simulink model "moon_riders"  (R2023a)
settings: Solver=FixedStepDiscrete  StartTime=0.0  StopTime=10.0  FixedStep=0.1  RelTol=1e-3
settings Model: Creator=Roger  LastModifiedBy=Roger
settings OptimizationCC: DefaultParameterBehavior=Inlined  EnhancedBackFolding=on  PassReuseOutputArgsAs=Individual arguments  ZeroExternalMemoryAtStartup=off  ZeroInternalMemoryAtStartup=off  OptimizeBlockOrder=speed  DifferentSizesBufferReuse=on  OptimizationCustomize=off  EfficientTunableParamExpr=on
settings DebuggingCC: ParameterTunabilityLossMsg=error
settings SFSimCC: MATLABDynamicMemAlloc=off
settings RTWCC: Description=Embedded Coder  SystemTargetFile=ert.tlc  TemplateMakefile=ert_default_tmf  GenerateReport=on  Toolchain=MinGW64 | CMake/gmake (64-bit Windows)  BuildConfiguration=Release  LaunchReport=on
settings CodeAppCC: ForceParamTrailComments=on  IgnoreCustomStorageClasses=off  OperatorAnnotations=on  SimulinkDataObjDesc=on  SFDataObjDesc=on  InsertBlockDesc=on
settings ERTTargetCC: TargetLangStandard=C99 (ISO)  GenerateSampleERTMain=on  InlinedParameterPlacement=NonHierarchical  ERTCustomFileTemplate=example_file_process.tlc

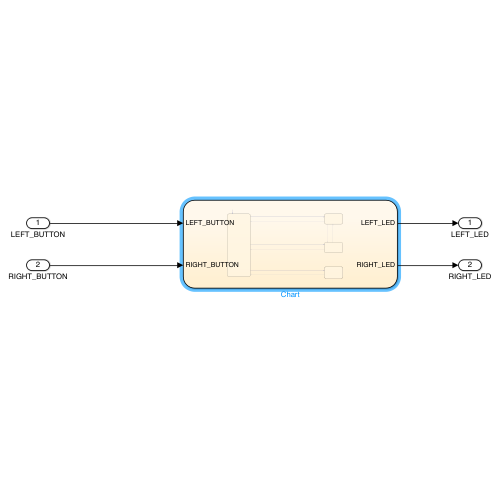
[thumbnail: Simulink's stored preview of the top-level diagram]
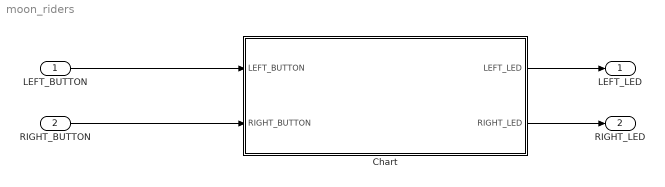
== system moon_riders ==
  LEFT_BUTTON : Inport
  "RIGHT_BUTTON " : Inport  Port=2
  Chart : Stateflow chart  TreatAsAtomicUnit=on
  LEFT_LED : Outport
  RIGHT_LED : Outport  Port=2
  wires:
  LEFT_BUTTON/1 -> Chart/1(LEFT_BUTTON)
  "RIGHT_BUTTON "/1 -> Chart/2(RIGHT_BUTTON)
  Chart/1(LEFT_LED) -> LEFT_LED/1
  Chart/2(RIGHT_LED) -> RIGHT_LED/1

== stateflow chart moon_riders/Chart ==
  state Idle
    entry:
    LEFT_LED = 0;
    RIGHT_LED = 0;
  state Left_Blinking
    entry:
    LEFT_LED = 1;
    RIGHT_LED = 0;
  state Right_Blinking
    entry:
    LEFT_LED = 0;
    RIGHT_LED = 1;
  state Hazard_Blinking
    entry:
    LEFT_LED = 1;
    RIGHT_LED = 1;
  (default) -> Idle
  Idle -> Left_Blinking [order 2] : [LEFT_BUTTON == 1]
  Left_Blinking -> Idle [order 2] : [LEFT_BUTTON == 1 && LEFT_LED==1]
  Left_Blinking -> Right_Blinking [order 1] : [RIGHT_BUTTON == 1&&LEFT_LED==1]
  Right_Blinking -> Left_Blinking [order 1] : [LEFT_BUTTON == 1&&RIGHT_LED==1]
  Idle -> Right_Blinking [order 3] : [RIGHT_BUTTON == 1 ]
  Right_Blinking -> Idle [order 2] : [RIGHT_BUTTON == 1&& RIGHT_LED == 1]
  Idle -> Hazard_Blinking [order 1] : [LEFT_BUTTON == 1 && RIGHT_BUTTON == 1]
  Hazard_Blinking -> Idle : [LEFT_BUTTON == 1 || RIGHT_BUTTON == 1]
  data: LEFT_BUTTON input; RIGHT_BUTTON input; LEFT_LED output; RIGHT_LED output
